simulink model "waterlevelcontroller_with_PID"  (R2024b)
settings: Solver=VariableStepAuto  StartTime=0.0  StopTime=1000  RelTol=1e-3
libraries: slpidlib x1
settings Model: Creator=Yasara  LastModifiedBy=Yasara

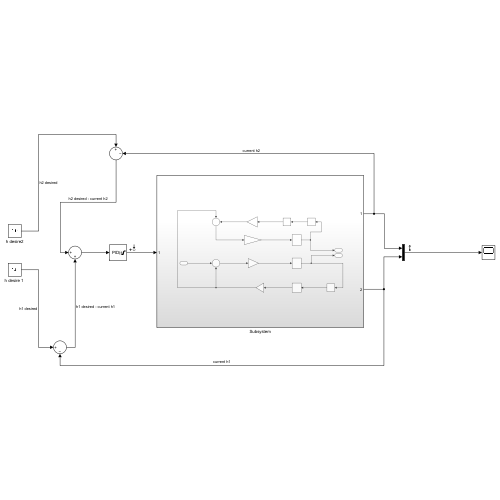
[thumbnail: Simulink's stored preview of the top-level diagram]
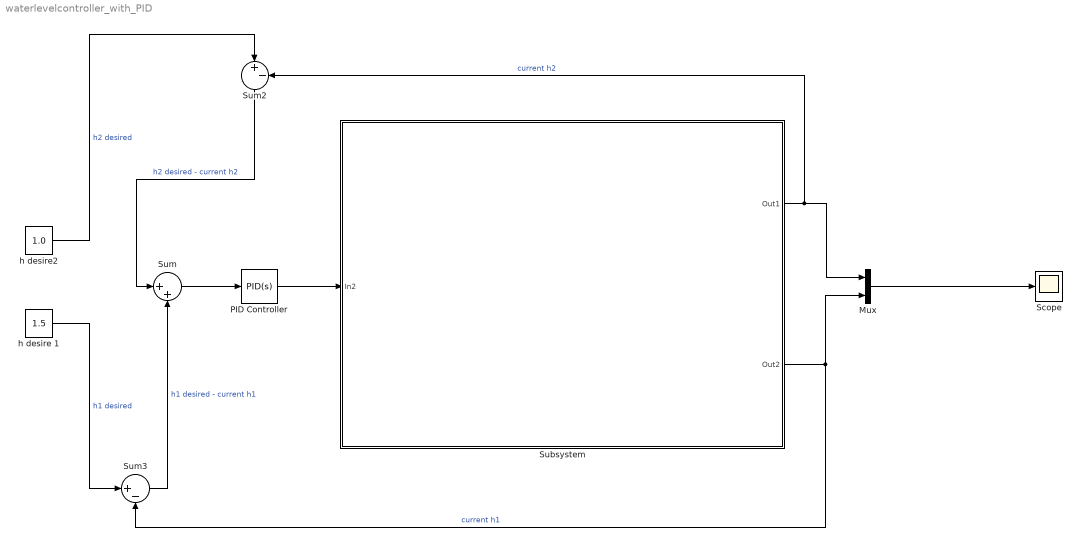
== system waterlevelcontroller_with_PID ==
  Mux : Mux  Inputs=2
  PID Controller : slpidlib/PID Controller  Controller=PID  Form=Parallel  TimeDomain=Continuous-time  UseExternalTs=off  SampleTime=-1  IntegratorMethod=Forward Euler  FilterMethod=Forward Euler  ControllerParametersSource=internal  P=8.0  I=0.8  UseKiTs=off  D=0.3  UseExternalDerivativeSource=off  N=50  UseFilter=on  TunerSelectOption=Transfer Function Based (PID Tuner App)  InitialConditionSource=internal  InitialConditionForIntegrator=0  InitialConditionForFilter=0  DifferentiatorICPrevScaledInput=0  ExternalReset=none  TrackingMode=off  Kt=1  LimitOutput=on  SatLimitsSource=internal  UpperSaturationLimit=5  LowerSaturationLimit=0  LinearizeAsGain=on  AntiWindupMode=back-calculation  Kb=1  LimitIntegrator=off  UpperIntegratorSaturationLimit=inf  LowerIntegratorSaturationLimit=-inf  POutMin=[]  POutMax=[]  IOutMin=[]  IOutMax=[]  DOutMin=[]  DOutMax=[]  NOutMin=[]  NOutMax=[]  SumOutMin=[]  SumOutMax=[]  SaturationOutMin=[]  SaturationOutMax=[]  PParamMin=[]  PParamMax=[]  IParamMin=[]  IParamMax=[]  DParamMin=[]  DParamMax=[]  NParamMin=[]  NParamMax=[]  KbParamMin=[]  KbParamMax=[]  KtParamMin=[]  KtParamMax=[]  KbOutMin=[]  KbOutMax=[]  KtOutMin=[]  KtOutMax=[]  IntegratorOutMin=[]  IntegratorOutMax=[]  FilterOutMin=[]  FilterOutMax=[]  SumI1OutMin=[]  SumI1OutMax=[]  SumI2OutMin=[]  SumI2OutMax=[]  SumI3OutMin=[]  SumI3OutMax=[]  SumI4OutMin=[]  SumI4OutMax=[]  SumDOutMin=[]  SumDOutMax=[]  DifferentiatorOutMin=[]  DifferentiatorOutMax=[]  FilterDiffOutCoefMin=[]  FilterDiffOutCoefMax=[]  ReciprocalOutMin=[]  ReciprocalOutMax=[]  SumDenOutMin=[]  SumDenOutMax=[]  SumNumOutMin=[]  SumNumOutMax=[]  DivideOutMin=[]  DivideOutMax=[]  UdiffTsProdOutMin=[]  UdiffTsProdOutMax=[]  NTsProdOutMin=[]  NTsProdOutMax=[]  UintegralTsProdOutMin=[]  UintegralTsProdOutMax=[]  UngainTsProdOutMin=[]  UngainTsProdOutMax=[]  ClampingZeroOutDataTypeStr=Inherit: Inherit via back propagation  ClampingZeroOutMin=[]  ClampingZeroOutMax=[]  FilterDenConstantOutDataTypeStr=Inherit: Inherit via back propagation  FilterDenConstantOutMin=[]  FilterDenConstantOutMax=[]  PCopyOutDataTypeStr=Inherit: Inherit via back propagation  PCopyOutMin=[]  PCopyOutMax=[]  NCopyOutDataTypeStr=Inherit: Inherit via back propagation  NCopyOutMin=[]  NCopyOutMax=[]  IntegratorContinuousStateAttributes=''  IntegratorStateMustResolveToSignalObject=off  IntegratorRTWStateStorageClass=Auto  FilterContinuousStateAttributes=''  FilterStateMustResolveToSignalObject=off  FilterRTWStateStorageClass=Auto  ParallelPVariant=InternalParameters  IdealPVariant=Disabled  IVariant=InternalParameters  DVariant=InternalParameters  IntegratorVariant=Continuous  SatVariant=Enabled  AWVariant=BackCalculation  PCopyVariant=Disabled  TRVariant=Disabled  FdbkBlocksVariant=Forward  IdealPFdbkVariant=Disabled  SatFdbkVariant=Disabled  DerivativeFilterVariant=ContFilter  NVariant=InternalParameters  NCopyVariant=Disabled  FilterICVariant=InternalICsFilter  IntegratorICVariant=InternalICs  ExternalResetVariant=Disabled  TRSumVariant=Passthrough  SumFdbkVariant=Disabled  SumVariant=Sum_PID  TsampFilterVariant=InternalTs  TsampNgainVariant=Passthrough  TsampIntegralVariant=Disabled_SignalSpec  ExternalSaturationOutDataTypeStr=Inherit: Same as second input  DerivativeSourceVariant=ErrorSignal  PreIntVariant=InternalPreInt
  Scope : Scope
  Subsystem : Subsystem
  Sum : Sum  Inputs=|++
  Sum2 : Sum  Inputs=|+-
  Sum3 : Sum  Inputs=|+-
  "h desire 1 " : Constant  Value=1.5
  h desire2 : Constant  Value=1.0
  wires:
  h desire2/1 -> Sum2/1  "h2 desired"
  "h desire 1 "/1 -> Sum3/1  "h1 desired"
  PID Controller/1 -> Subsystem/1(In2)
  Subsystem/2(Out2) -> Sum3/2, Mux/2  "current h1"
  Subsystem/1(Out1) -> Mux/1, Sum2/2  "current h2"
  Mux/1 -> Scope/1
  Sum2/1 -> Sum/1  "h2 desired - current h2"
  Sum3/1 -> Sum/2  "h1 desired - current h1"
  Sum/1 -> PID Controller/1

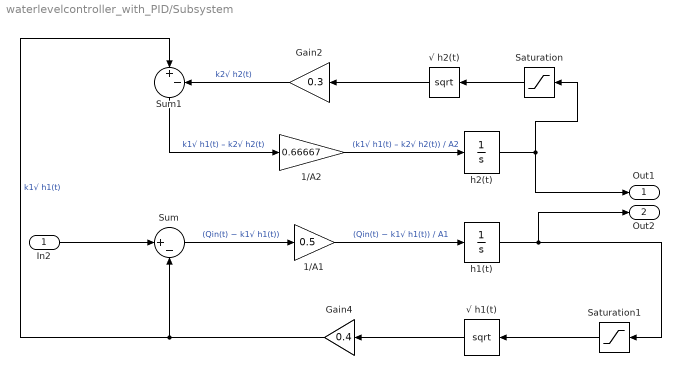
== system waterlevelcontroller_with_PID/Subsystem ==
  In2 : Inport
  1/A1 : Gain  Gain=0.5
  1/A2 : Gain  Gain=0.66667
  Gain2 : Gain  Gain=0.3
  Gain4 : Gain  Gain=0.4
  Saturation : Saturate  UpperLimit=inf  LowerLimit=0
  Saturation1 : Saturate  UpperLimit=inf  LowerLimit=0
  Sum : Sum  Inputs=|+-
  Sum1 : Sum  Inputs=|+-
  h1(t) : Integrator
  h2(t) : Integrator
  √ h1(t) : Sqrt
  √ h2(t) : Sqrt
  Out1 : Outport
  Out2 : Outport  Port=2
  wires:
  √ h1(t)/1 -> Gain4/1
  Sum/1 -> 1/A1/1  "(Qin(t) − k1√ h1(t))"
  √ h2(t)/1 -> Gain2/1
  1/A1/1 -> h1(t)/1  "(Qin(t) − k1√ h1(t)) / A1"
  Gain2/1 -> Sum1/2  "k2√ h2(t)"
  1/A2/1 -> h2(t)/1  "(k1√ h1(t) – k2√ h2(t)) / A2"
  In2/1 -> Sum/1
  Gain4/1 -> Sum/2, Sum1/1  "k1√ h1(t)"
  h2(t)/1 -> Saturation/1, Out1/1
  h1(t)/1 -> Saturation1/1, Out2/1
  Sum1/1 -> 1/A2/1  "k1√ h1(t) – k2√ h2(t)"
  Saturation/1 -> √ h2(t)/1
  Saturation1/1 -> √ h1(t)/1
